simulink library "halin"  (R2021b)
settings: Solver=VariableStepAuto  StartTime=0.0  StopTime=10.0  RelTol=1e-3
undefined symbols (not defined in the file): KHAL_CAN1ABM1E2E_flg, KHAL_CAN1ESC1E2E_flg, KHAL_CAN1ESC5E2E_flg, KHAL_CAN1ESC7E2E_flg, KHAL_CAN1FCM2E2E_flg, KHAL_CAN1FCM3E2E_flg, KHAL_CAN1FCM4E2E_flg, KHAL_CAN3BMS1E2E_flg, KHAL_CAN3BMS6E2E_flg, KHAL_CAN3CCU1E2E_flg, KHAL_CAN3CCU2E2E_flg, KHAL_CAN3MCUF1E2E_flg, KHAL_CAN3MCUR1E2E_flg, KHAL_CAN3Shifter1E2E_flg, TRUE
libraries: simulink x420, FVT_lib x149, hcu_lib x49
(part 4 of 14)

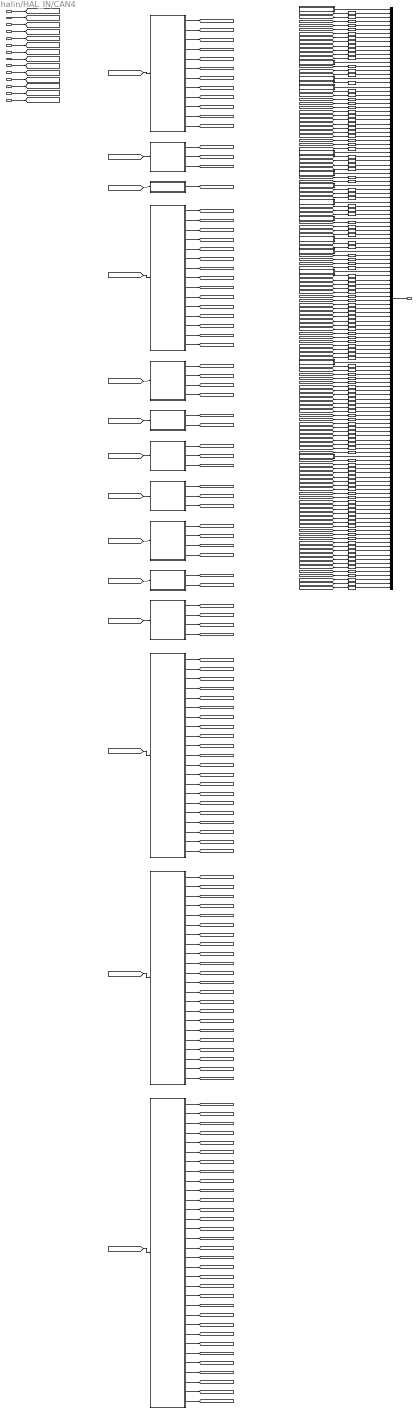
== system halin/HAL_IN/CAN4 ==
  DT_CAN4_SG_DKC1 : Inport
  DT_CAN4_SG_DKC2 : Inport  Port=2
  DT_CAN4_SG_GW_ZDR_PTG1 : Inport  Port=3
  DT_CAN4_SG_GW_ZoneDR1 : Inport  Port=4
  DT_CAN4_SG_GW_ZoneDR2 : Inport  Port=5
  DT_CAN4_SG_GW_ZoneDR3 : Inport  Port=6
  DT_CAN4_SG_GW_ZoneDR4 : Inport  Port=7
  DT_CAN4_SG_GW_ZoneDR6 : Inport  Port=8
  DT_CAN4_SG_GW_ZoneFR1 : Inport  Port=9
  DT_CAN4_SG_GW_ZoneFR2 : Inport  Port=10
  DT_CAN4_SG_Zone_Dr_SCP : Inport  Port=11
  DT_CAN4_SG_Zone_Dr_THCM : Inport  Port=12
  DT_CAN4_SG_Zone_Dr_VCU : Inport  Port=13
  DT_CAN4_SG_Zone_Fr_THCM : Inport  Port=14
  DKC1 : Subsystem
  DKC2 : Subsystem
  GW_ZDR_PTG1 : Subsystem
  GW_ZoneDR1 : Subsystem
  GW_ZoneDR2 : Subsystem
  GW_ZoneDR3 : Subsystem
  GW_ZoneDR4 : Subsystem
  GW_ZoneDR6 : Subsystem
  GW_ZoneFR1 : Subsystem
  GW_ZoneFR2 : Subsystem
  UnitConverter{,1..8,10,15,17..18,20..22,26,39,50,52..53,55,57,59,61,63,65,67,69,71,73,76,79..81,90,92,94..96,98,100..105,107,109,111,113,115,117,119,121..125,127} (60 alike) : DataTypeConversion  OutDataTypeStr=uint8
  UnitConverter{27..28,35..38,40..44,47,51,54,56,58,60,62,64,66,68,70,72,74..75,77..78,85..86,88..89,91,97,99,106,108,110,112,114,116,118,120,126} (43 alike) : DataTypeConversion  OutDataTypeStr=single
  UnitConverter{9,11,16,19,23..25,29..34,45..46,48..49,82..84,87,93} (22 alike) : DataTypeConversion  OutDataTypeStr=boolean
  UnitConverter12 : DataTypeConversion  OutDataTypeStr=uint64
  UnitConverter13 : DataTypeConversion  OutDataTypeStr=uint64
  UnitConverter14 : DataTypeConversion  OutDataTypeStr=uint64
  VHAL_CANMsgInvalidDKC1_flg : Subsystem  AncestorBlock=FVT_lib/hal/MsgTimeoutJudge_CAN_AUTOSAR
      mask help: MeasumentTrigerEvent
      mask Display: fprintf('MsgTimeoutJudge_CAN\nAUTOSAR');
  VHAL_CANMsgInvalidDKC2_flg : Subsystem  AncestorBlock=FVT_lib/hal/MsgTimeoutJudge_CAN_AUTOSAR
      mask help: MeasumentTrigerEvent
      mask Display: fprintf('MsgTimeoutJudge_CAN\nAUTOSAR');
  VHAL_CANMsgInvalidGWZDRPTG1_flg : Subsystem  AncestorBlock=FVT_lib/hal/MsgTimeoutJudge_CAN_AUTOSAR
      mask help: MeasumentTrigerEvent
      mask Display: fprintf('MsgTimeoutJudge_CAN\nAUTOSAR');
  VHAL_CANMsgInvalidGWZoneDR1_flg : Subsystem  AncestorBlock=FVT_lib/hal/MsgTimeoutJudge_CAN_AUTOSAR
      mask help: MeasumentTrigerEvent
      mask Display: fprintf('MsgTimeoutJudge_CAN\nAUTOSAR');
  VHAL_CANMsgInvalidGWZoneDR2_flg : Subsystem  AncestorBlock=FVT_lib/hal/MsgTimeoutJudge_CAN_AUTOSAR
      mask help: MeasumentTrigerEvent
      mask Display: fprintf('MsgTimeoutJudge_CAN\nAUTOSAR');
  VHAL_CANMsgInvalidGWZoneDR3_flg : Subsystem  AncestorBlock=FVT_lib/hal/MsgTimeoutJudge_CAN_AUTOSAR
      mask help: MeasumentTrigerEvent
      mask Display: fprintf('MsgTimeoutJudge_CAN\nAUTOSAR');
  VHAL_CANMsgInvalidGWZoneDR4_flg : Subsystem  AncestorBlock=FVT_lib/hal/MsgTimeoutJudge_CAN_AUTOSAR
      mask help: MeasumentTrigerEvent
      mask Display: fprintf('MsgTimeoutJudge_CAN\nAUTOSAR');
  VHAL_CANMsgInvalidGWZoneDR6_flg : Subsystem  AncestorBlock=FVT_lib/hal/MsgTimeoutJudge_CAN_AUTOSAR
      mask help: MeasumentTrigerEvent
      mask Display: fprintf('MsgTimeoutJudge_CAN\nAUTOSAR');
  VHAL_CANMsgInvalidGWZoneFR1_flg : Subsystem  AncestorBlock=FVT_lib/hal/MsgTimeoutJudge_CAN_AUTOSAR
      mask help: MeasumentTrigerEvent
      mask Display: fprintf('MsgTimeoutJudge_CAN\nAUTOSAR');
  VHAL_CANMsgInvalidGWZoneFR2_flg : Subsystem  AncestorBlock=FVT_lib/hal/MsgTimeoutJudge_CAN_AUTOSAR
      mask help: MeasumentTrigerEvent
      mask Display: fprintf('MsgTimeoutJudge_CAN\nAUTOSAR');
  VHAL_CANMsgInvalidZoneDrSCP_flg : Subsystem  AncestorBlock=FVT_lib/hal/MsgTimeoutJudge_CAN_AUTOSAR
      mask help: MeasumentTrigerEvent
      mask Display: fprintf('MsgTimeoutJudge_CAN\nAUTOSAR');
  VHAL_CANMsgInvalidZoneDrTHCM_flg : Subsystem  AncestorBlock=FVT_lib/hal/MsgTimeoutJudge_CAN_AUTOSAR
      mask help: MeasumentTrigerEvent
      mask Display: fprintf('MsgTimeoutJudge_CAN\nAUTOSAR');
  VHAL_CANMsgInvalidZoneDrVCU_flg : Subsystem  AncestorBlock=FVT_lib/hal/MsgTimeoutJudge_CAN_AUTOSAR
      mask help: MeasumentTrigerEvent
      mask Display: fprintf('MsgTimeoutJudge_CAN\nAUTOSAR');
  VHAL_CANMsgInvalidZoneFrTHCM_flg : Subsystem  AncestorBlock=FVT_lib/hal/MsgTimeoutJudge_CAN_AUTOSAR
      mask help: MeasumentTrigerEvent
      mask Display: fprintf('MsgTimeoutJudge_CAN\nAUTOSAR');
  Zone_Dr_SCP : Subsystem
  Zone_Dr_THCM : Subsystem
  Zone_Dr_VCU : Subsystem
  Zone_Fr_THCM : Subsystem
  bus_creator : BusCreator  Inputs=142
  HAL_CAN4_outputs : Outport
  wires:
  DT_CAN4_SG_DKC1/1 -> [DT_CAN4_SG_DKC1]
  DT_CAN4_SG_DKC2/1 -> [DT_CAN4_SG_DKC2]
  DT_CAN4_SG_GW_ZDR_PTG1/1 -> [DT_CAN4_SG_GW_ZDR_PTG1]
  DT_CAN4_SG_GW_ZoneDR1/1 -> [DT_CAN4_SG_GW_ZoneDR1]
  DT_CAN4_SG_GW_ZoneDR2/1 -> [DT_CAN4_SG_GW_ZoneDR2]
  DT_CAN4_SG_GW_ZoneDR3/1 -> [DT_CAN4_SG_GW_ZoneDR3]
  DT_CAN4_SG_GW_ZoneDR4/1 -> [DT_CAN4_SG_GW_ZoneDR4]
  DT_CAN4_SG_GW_ZoneDR6/1 -> [DT_CAN4_SG_GW_ZoneDR6]
  DT_CAN4_SG_GW_ZoneFR1/1 -> [DT_CAN4_SG_GW_ZoneFR1]
  DT_CAN4_SG_GW_ZoneFR2/1 -> [DT_CAN4_SG_GW_ZoneFR2]
  DT_CAN4_SG_Zone_Dr_SCP/1 -> [DT_CAN4_SG_Zone_Dr_SCP]
  DT_CAN4_SG_Zone_Dr_THCM/1 -> [DT_CAN4_SG_Zone_Dr_THCM]
  DT_CAN4_SG_Zone_Dr_VCU/1 -> [DT_CAN4_SG_Zone_Dr_VCU]
  DT_CAN4_SG_Zone_Fr_THCM/1 -> [DT_CAN4_SG_Zone_Fr_THCM]
  [DT_CAN4_SG_DKC1] -> DKC1/1(DT_CAN4_SG_DKC1)
  [DT_CAN4_SG_DKC2] -> DKC2/1(DT_CAN4_SG_DKC2)
  [DT_CAN4_SG_GW_ZDR_PTG1] -> GW_ZDR_PTG1/1(DT_CAN4_SG_GW_ZDR_PTG1)
  [DT_CAN4_SG_GW_ZoneDR1] -> GW_ZoneDR1/1(DT_CAN4_SG_GW_ZoneDR1)
  [DT_CAN4_SG_GW_ZoneDR2] -> GW_ZoneDR2/1(DT_CAN4_SG_GW_ZoneDR2)
  [DT_CAN4_SG_GW_ZoneDR3] -> GW_ZoneDR3/1(DT_CAN4_SG_GW_ZoneDR3)
  [DT_CAN4_SG_GW_ZoneDR4] -> GW_ZoneDR4/1(DT_CAN4_SG_GW_ZoneDR4)
  [DT_CAN4_SG_GW_ZoneDR6] -> GW_ZoneDR6/1(DT_CAN4_SG_GW_ZoneDR6)
  [DT_CAN4_SG_GW_ZoneFR1] -> GW_ZoneFR1/1(DT_CAN4_SG_GW_ZoneFR1)
  [DT_CAN4_SG_GW_ZoneFR2] -> GW_ZoneFR2/1(DT_CAN4_SG_GW_ZoneFR2)
  [DT_CAN4_SG_Zone_Dr_SCP] -> Zone_Dr_SCP/1(DT_CAN4_SG_Zone_Dr_SCP)
  [DT_CAN4_SG_Zone_Dr_THCM] -> Zone_Dr_THCM/1(DT_CAN4_SG_Zone_Dr_THCM)
  [DT_CAN4_SG_Zone_Dr_VCU] -> Zone_Dr_VCU/1(DT_CAN4_SG_Zone_Dr_VCU)
  [DT_CAN4_SG_Zone_Fr_THCM] -> Zone_Fr_THCM/1(DT_CAN4_SG_Zone_Fr_THCM)
  bus_creator/1 -> HAL_CAN4_outputs/1
  VHAL_CANMsgInvalidDKC1_flg/1(Out) -> bus_creator/1
  DKC1/1(VHAL_DKCReVehData_enum) -> [VHAL_DKCReVehData_enum]
  UnitConverter/1 -> bus_creator/2  "VHAL_DKCReVehData_enum"
  [VHAL_DKCReVehData_enum] -> UnitConverter/1
  DKC1/2(VHAL_DKCRemotePW_enum) -> [VHAL_DKCRemotePW_enum]
  UnitConverter1/1 -> bus_creator/3  "VHAL_DKCRemotePW_enum"
  [VHAL_DKCRemotePW_enum] -> UnitConverter1/1
  DKC1/3(VHAL_PCommandToBCM_enum) -> [VHAL_PCommandToBCM_enum]
  UnitConverter2/1 -> bus_creator/4  "VHAL_PCommandToBCM_enum"
  [VHAL_PCommandToBCM_enum] -> UnitConverter2/1
  DKC1/4(VHAL_PCommandToPTG_enum) -> [VHAL_PCommandToPTG_enum]
  UnitConverter3/1 -> bus_creator/5  "VHAL_PCommandToPTG_enum"
  [VHAL_PCommandToPTG_enum] -> UnitConverter3/1
  DKC1/5(VHAL_PDKeyAreaLockUnlock_enum) -> [VHAL_PDKeyAreaLockUnlock_enum]
  UnitConverter4/1 -> bus_creator/6  "VHAL_PDKeyAreaLockUnlock_enum"
  [VHAL_PDKeyAreaLockUnlock_enum] -> UnitConverter4/1
  DKC1/6(VHAL_PDKeyAreaPS_enum) -> [VHAL_PDKeyAreaPS_enum]
  UnitConverter5/1 -> bus_creator/7  "VHAL_PDKeyAreaPS_enum"
  [VHAL_PDKeyAreaPS_enum] -> UnitConverter5/1
  DKC1/7(VHAL_PDKeyAreaPTG_enum) -> [VHAL_PDKeyAreaPTG_enum]
  UnitConverter6/1 -> bus_creator/8  "VHAL_PDKeyAreaPTG_enum"
  [VHAL_PDKeyAreaPTG_enum] -> UnitConverter6/1
  DKC1/8(VHAL_PDKeyWelcome_enum) -> [VHAL_PDKeyWelcome_enum]
  UnitConverter7/1 -> bus_creator/9  "VHAL_PDKeyWelcome_enum"
  [VHAL_PDKeyWelcome_enum] -> UnitConverter7/1
  DKC1/9(VHAL_PDkeyShowIVI_enum) -> [VHAL_PDkeyShowIVI_enum]
  UnitConverter8/1 -> bus_creator/10  "VHAL_PDkeyShowIVI_enum"
  [VHAL_PDkeyShowIVI_enum] -> UnitConverter8/1
  DKC1/10(VHAL_PKeyMiss_flg) -> [VHAL_PKeyMiss_flg]
  UnitConverter9/1 -> bus_creator/11  "VHAL_PKeyMiss_flg"
  [VHAL_PKeyMiss_flg] -> UnitConverter9/1
  DKC1/11(VHAL_PKeyMode_enum) -> [VHAL_PKeyMode_enum]
  UnitConverter10/1 -> bus_creator/12  "VHAL_PKeyMode_enum"
  [VHAL_PKeyMode_enum] -> UnitConverter10/1
  DKC1/12(VHAL_PUIDLowPower_flg) -> [VHAL_PUIDLowPower_flg]
  UnitConverter11/1 -> bus_creator/13  "VHAL_PUIDLowPower_flg"
  [VHAL_PUIDLowPower_flg] -> UnitConverter11/1
  VHAL_CANMsgInvalidDKC2_flg/1(Out) -> bus_creator/14
  DKC2/1(VHAL_EncryptionDATA063_enum) -> [VHAL_EncryptionDATA063_enum]
  UnitConverter12/1 -> bus_creator/15  "VHAL_EncryptionDATA063_enum"
  [VHAL_EncryptionDATA063_enum] -> UnitConverter12/1
  DKC2/2(VHAL_EncryptionDATA64127_enum) -> [VHAL_EncryptionDATA64127_enum]
  UnitConverter13/1 -> bus_creator/16  "VHAL_EncryptionDATA64127_enum"
  [VHAL_EncryptionDATA64127_enum] -> UnitConverter13/1
  DKC2/3(VHAL_RandomNumberX_enum) -> [VHAL_RandomNumberX_enum]
  UnitConverter14/1 -> bus_creator/17  "VHAL_RandomNumberX_enum"
  [VHAL_RandomNumberX_enum] -> UnitConverter14/1
  VHAL_CANMsgInvalidGWZDRPTG1_flg/1(Out) -> bus_creator/18
  GW_ZDR_PTG1/1(VHAL_PTGRDILSta_enum) -> [VHAL_PTGRDILSta_enum]
  UnitConverter15/1 -> bus_creator/19  "VHAL_PTGRDILSta_enum"
  [VHAL_PTGRDILSta_enum] -> UnitConverter15/1
  VHAL_CANMsgInvalidGWZoneDR1_flg/1(Out) -> bus_creator/20
  GW_ZoneDR1/1(VHAL_CSWDimSw_flg) -> [VHAL_CSWDimSw_flg]
  UnitConverter16/1 -> bus_creator/21  "VHAL_CSWDimSw_flg"
  [VHAL_CSWDimSw_flg] -> UnitConverter16/1
  GW_ZoneDR1/2(VHAL_CSWFWasSwSta_enum) -> [VHAL_CSWFWasSwSta_enum]
  UnitConverter17/1 -> bus_creator/22  "VHAL_CSWFWasSwSta_enum"
  [VHAL_CSWFWasSwSta_enum] -> UnitConverter17/1
  GW_ZoneDR1/3(VHAL_CSWFWipSwSta_enum) -> [VHAL_CSWFWipSwSta_enum]
  UnitConverter18/1 -> bus_creator/23  "VHAL_CSWFWipSwSta_enum"
  [VHAL_CSWFWipSwSta_enum] -> UnitConverter18/1
  GW_ZoneDR1/4(VHAL_CSWPassSWSta_flg) -> [VHAL_CSWPassSWSta_flg]
  UnitConverter19/1 -> bus_creator/24  "VHAL_CSWPassSWSta_flg"
  [VHAL_CSWPassSWSta_flg] -> UnitConverter19/1
  GW_ZoneDR1/5(VHAL_CSWRWasSWSta_enum) -> [VHAL_CSWRWasSWSta_enum]
  UnitConverter20/1 -> bus_creator/25  "VHAL_CSWRWasSWSta_enum"
  [VHAL_CSWRWasSWSta_enum] -> UnitConverter20/1
  GW_ZoneDR1/6(VHAL_CSWRWipIntSwSta_enum) -> [VHAL_CSWRWipIntSwSta_enum]
  UnitConverter21/1 -> bus_creator/26  "VHAL_CSWRWipIntSwSta_enum"
  [VHAL_CSWRWipIntSwSta_enum] -> UnitConverter21/1
  GW_ZoneDR1/7(VHAL_CSWTurnSwSta_enum) -> [VHAL_CSWTurnSwSta_enum]
  UnitConverter22/1 -> bus_creator/27  "VHAL_CSWTurnSwSta_enum"
  [VHAL_CSWTurnSwSta_enum] -> UnitConverter22/1
  GW_ZoneDR1/8(VHAL_DrLockSta_flg) -> [VHAL_DrLockSta_flg]
  UnitConverter23/1 -> bus_creator/28  "VHAL_DrLockSta_flg"
  [VHAL_DrLockSta_flg] -> UnitConverter23/1
  GW_ZoneDR1/9(VHAL_MIRRORFOLDSW_flg) -> [VHAL_MIRRORFOLDSW_flg]
  UnitConverter24/1 -> bus_creator/29  "VHAL_MIRRORFOLDSW_flg"
  [VHAL_MIRRORFOLDSW_flg] -> UnitConverter24/1
  GW_ZoneDR1/10(VHAL_RLSLampSta_flg) -> [VHAL_RLSLampSta_flg]
  UnitConverter25/1 -> bus_creator/30  "VHAL_RLSLampSta_flg"
  [VHAL_RLSLampSta_flg] -> UnitConverter25/1
  GW_ZoneDR1/11(VHAL_RLSRainSnrWiperCmd_enum) -> [VHAL_RLSRainSnrWiperCmd_enum]
  UnitConverter26/1 -> bus_creator/31  "VHAL_RLSRainSnrWiperCmd_enum"
  [VHAL_RLSRainSnrWiperCmd_enum] -> UnitConverter26/1
  GW_ZoneDR1/12(VHAL_RLTurnLampC_mA) -> [VHAL_RLTurnLampC_mA]
  UnitConverter27/1 -> bus_creator/32  "VHAL_RLTurnLampC_mA"
  [VHAL_RLTurnLampC_mA] -> UnitConverter27/1
  GW_ZoneDR1/13(VHAL_RRTurnLampC_mA) -> [VHAL_RRTurnLampC_mA]
  UnitConverter28/1 -> bus_creator/33  "VHAL_RRTurnLampC_mA"
  [VHAL_RRTurnLampC_mA] -> UnitConverter28/1
  GW_ZoneDR1/14(VHAL_RWiperAS_flg) -> [VHAL_RWiperAS_flg]
  UnitConverter29/1 -> bus_creator/34  "VHAL_RWiperAS_flg"
  [VHAL_RWiperAS_flg] -> UnitConverter29/1
  GW_ZoneDR1/15(VHAL_RWiperProtection_flg) -> [VHAL_RWiperProtection_flg]
  UnitConverter30/1 -> bus_creator/35  "VHAL_RWiperProtection_flg"
  [VHAL_RWiperProtection_flg] -> UnitConverter30/1
  VHAL_CANMsgInvalidGWZoneDR2_flg/1(Out) -> bus_creator/36
  GW_ZoneDR2/1(VHAL_SWCCANCELSta_flg) -> [VHAL_SWCCANCELSta_flg]
  UnitConverter31/1 -> bus_creator/37  "VHAL_SWCCANCELSta_flg"
  [VHAL_SWCCANCELSta_flg] -> UnitConverter31/1
  GW_ZoneDR2/2(VHAL_SWCResUpSta_flg) -> [VHAL_SWCResUpSta_flg]
  UnitConverter32/1 -> bus_creator/38  "VHAL_SWCResUpSta_flg"
  [VHAL_SWCResUpSta_flg] -> UnitConverter32/1
  GW_ZoneDR2/3(VHAL_SWCSetdownSta_flg) -> [VHAL_SWCSetdownSta_flg]
  UnitConverter33/1 -> bus_creator/39  "VHAL_SWCSetdownSta_flg"
  [VHAL_SWCSetdownSta_flg] -> UnitConverter33/1
  GW_ZoneDR2/4(VHAL_SWCmodeSta_flg) -> [VHAL_SWCmodeSta_flg]
  UnitConverter34/1 -> bus_creator/40  "VHAL_SWCmodeSta_flg"
  [VHAL_SWCmodeSta_flg] -> UnitConverter34/1
  VHAL_CANMsgInvalidGWZoneDR3_flg/1(Out) -> bus_creator/41
  GW_ZoneDR3/1(VHAL_LDrvValWdwOpened_pct) -> [VHAL_LDrvValWdwOpened_pct]
  UnitConverter35/1 -> bus_creator/42  "VHAL_LDrvValWdwOpened_pct"
  [VHAL_LDrvValWdwOpened_pct] -> UnitConverter35/1
  GW_ZoneDR3/2(VHAL_LPasValWdwOpened_pct) -> [VHAL_LPasValWdwOpened_pct]
  UnitConverter36/1 -> bus_creator/43  "VHAL_LPasValWdwOpened_pct"
  [VHAL_LPasValWdwOpened_pct] -> UnitConverter36/1
  VHAL_CANMsgInvalidGWZoneDR4_flg/1(Out) -> bus_creator/44
  GW_ZoneDR4/1(VHAL_LRLDValWdwOpened_pct) -> [VHAL_LRLDValWdwOpened_pct]
  UnitConverter37/1 -> bus_creator/45  "VHAL_LRLDValWdwOpened_pct"
  [VHAL_LRLDValWdwOpened_pct] -> UnitConverter37/1
  GW_ZoneDR4/2(VHAL_LRRDValWdwOpened_pct) -> [VHAL_LRRDValWdwOpened_pct]
  UnitConverter38/1 -> bus_creator/46  "VHAL_LRRDValWdwOpened_pct"
  [VHAL_LRRDValWdwOpened_pct] -> UnitConverter38/1
  GW_ZoneDR4/3(VHAL_PTGInnerSW2_enum) -> [VHAL_PTGInnerSW2_enum]
  UnitConverter39/1 -> bus_creator/47  "VHAL_PTGInnerSW2_enum"
  [VHAL_PTGInnerSW2_enum] -> UnitConverter39/1
  VHAL_CANMsgInvalidGWZoneDR6_flg/1(Out) -> bus_creator/48
  GW_ZoneDR6/1(VHAL_FrntPTCRearLeActHeatPwr_W) -> [VHAL_FrntPTCRearLeActHeatPwr_W]
  UnitConverter40/1 -> bus_creator/49  "VHAL_FrntPTCRearLeActHeatPwr_W"
  [VHAL_FrntPTCRearLeActHeatPwr_W] -> UnitConverter40/1
  GW_ZoneDR6/2(VHAL_FrntPTCRearRiActHeatPwr_W) -> [VHAL_FrntPTCRearRiActHeatPwr_W]
  UnitConverter41/1 -> bus_creator/50  "VHAL_FrntPTCRearRiActHeatPwr_W"
  [VHAL_FrntPTCRearRiActHeatPwr_W] -> UnitConverter41/1
  GW_ZoneDR6/3(VHAL_FrntPTCRiActHeatPwr_W) -> [VHAL_FrntPTCRiActHeatPwr_W]
  UnitConverter42/1 -> bus_creator/51  "VHAL_FrntPTCRiActHeatPwr_W"
  [VHAL_FrntPTCRiActHeatPwr_W] -> UnitConverter42/1
  VHAL_CANMsgInvalidGWZoneFR1_flg/1(Out) -> bus_creator/52
  GW_ZoneFR1/1(VHAL_FLTurnLampC_mA) -> [VHAL_FLTurnLampC_mA]
  UnitConverter43/1 -> bus_creator/53  "VHAL_FLTurnLampC_mA"
  [VHAL_FLTurnLampC_mA] -> UnitConverter43/1
  GW_ZoneFR1/2(VHAL_FRTurnLampC_mA) -> [VHAL_FRTurnLampC_mA]
  UnitConverter44/1 -> bus_creator/54  "VHAL_FRTurnLampC_mA"
  [VHAL_FRTurnLampC_mA] -> UnitConverter44/1
  GW_ZoneFR1/3(VHAL_FWiperAS_flg) -> [VHAL_FWiperAS_flg]
  UnitConverter45/1 -> bus_creator/55  "VHAL_FWiperAS_flg"
  [VHAL_FWiperAS_flg] -> UnitConverter45/1
  GW_ZoneFR1/4(VHAL_FWiperProtection_flg) -> [VHAL_FWiperProtection_flg]
  UnitConverter46/1 -> bus_creator/56  "VHAL_FWiperProtection_flg"
  [VHAL_FWiperProtection_flg] -> UnitConverter46/1
  VHAL_CANMsgInvalidGWZoneFR2_flg/1(Out) -> bus_creator/57
  GW_ZoneFR2/1(VHAL_COMPStatorSpd_rpm) -> [VHAL_COMPStatorSpd_rpm]
  UnitConverter47/1 -> bus_creator/58  "VHAL_COMPStatorSpd_rpm"
  [VHAL_COMPStatorSpd_rpm] -> UnitConverter47/1
  GW_ZoneFR2/2(VHAL_CompProEN_flg) -> [VHAL_CompProEN_flg]
  UnitConverter48/1 -> bus_creator/59  "VHAL_CompProEN_flg"
  [VHAL_CompProEN_flg] -> UnitConverter48/1
  VHAL_CANMsgInvalidZoneDrSCP_flg/1(Out) -> bus_creator/60
  Zone_Dr_SCP/1(VHAL_DrSCPSysErrLmp_flg) -> [VHAL_DrSCPSysErrLmp_flg]
  UnitConverter49/1 -> bus_creator/61  "VHAL_DrSCPSysErrLmp_flg"
  [VHAL_DrSCPSysErrLmp_flg] -> UnitConverter49/1
  Zone_Dr_SCP/2(VHAL_RegenMode_enum) -> [VHAL_RegenMode_enum]
  UnitConverter50/1 -> bus_creator/62  "VHAL_RegenMode_enum"
  [VHAL_RegenMode_enum] -> UnitConverter50/1
  Zone_Dr_SCP/3(VHAL_SetSpd_kph) -> [VHAL_SetSpd_kph]
  UnitConverter51/1 -> bus_creator/63  "VHAL_SetSpd_kph"
  [VHAL_SetSpd_kph] -> UnitConverter51/1
  Zone_Dr_SCP/4(VHAL_ZoneSpdCtrlMode_enum) -> [VHAL_ZoneSpdCtrlMode_enum]
  UnitConverter52/1 -> bus_creator/64  "VHAL_ZoneSpdCtrlMode_enum"
  [VHAL_ZoneSpdCtrlMode_enum] -> UnitConverter52/1
  VHAL_CANMsgInvalidZoneDrTHCM_flg/1(Out) -> bus_creator/65
  Zone_Dr_THCM/1(VHAL_BlowerErr_enum) -> [VHAL_BlowerErr_enum]
  UnitConverter53/1 -> bus_creator/66  "VHAL_BlowerErr_enum"
  [VHAL_BlowerErr_enum] -> UnitConverter53/1
  Zone_Dr_THCM/2(VHAL_SolarL_W) -> [VHAL_SolarL_W]
  UnitConverter54/1 -> bus_creator/67  "VHAL_SolarL_W"
  [VHAL_SolarL_W] -> UnitConverter54/1
  Zone_Dr_THCM/3(VHAL_SolarLErr_enum) -> [VHAL_SolarLErr_enum]
  UnitConverter55/1 -> bus_creator/68  "VHAL_SolarLErr_enum"
  [VHAL_SolarLErr_enum] -> UnitConverter55/1
  Zone_Dr_THCM/4(VHAL_SolarR_W) -> [VHAL_SolarR_W]
  UnitConverter56/1 -> bus_creator/69  "VHAL_SolarR_W"
  [VHAL_SolarR_W] -> UnitConverter56/1
  Zone_Dr_THCM/5(VHAL_SolarRErr_enum) -> [VHAL_SolarRErr_enum]
  UnitConverter57/1 -> bus_creator/70  "VHAL_SolarRErr_enum"
  [VHAL_SolarRErr_enum] -> UnitConverter57/1
  Zone_Dr_THCM/6(VHAL_TFaceL_C) -> [VHAL_TFaceL_C]
  UnitConverter58/1 -> bus_creator/71  "VHAL_TFaceL_C"
  [VHAL_TFaceL_C] -> UnitConverter58/1
  Zone_Dr_THCM/7(VHAL_TFaceLErr_enum) -> [VHAL_TFaceLErr_enum]
  UnitConverter59/1 -> bus_creator/72  "VHAL_TFaceLErr_enum"
  [VHAL_TFaceLErr_enum] -> UnitConverter59/1
  Zone_Dr_THCM/8(VHAL_TFaceR_C) -> [VHAL_TFaceR_C]
  UnitConverter60/1 -> bus_creator/73  "VHAL_TFaceR_C"
  [VHAL_TFaceR_C] -> UnitConverter60/1
  Zone_Dr_THCM/9(VHAL_TFaceRErr_enum) -> [VHAL_TFaceRErr_enum]
  UnitConverter61/1 -> bus_creator/74  "VHAL_TFaceRErr_enum"
  [VHAL_TFaceRErr_enum] -> UnitConverter61/1
  Zone_Dr_THCM/10(VHAL_TFaceRr_C) -> [VHAL_TFaceRr_C]
  UnitConverter62/1 -> bus_creator/75  "VHAL_TFaceRr_C"
  [VHAL_TFaceRr_C] -> UnitConverter62/1
  Zone_Dr_THCM/11(VHAL_TFaceRrErr_enum) -> [VHAL_TFaceRrErr_enum]
  UnitConverter63/1 -> bus_creator/76  "VHAL_TFaceRrErr_enum"
  [VHAL_TFaceRrErr_enum] -> UnitConverter63/1
  Zone_Dr_THCM/12(VHAL_TFootL_C) -> [VHAL_TFootL_C]
  UnitConverter64/1 -> bus_creator/77  "VHAL_TFootL_C"
  [VHAL_TFootL_C] -> UnitConverter64/1
  Zone_Dr_THCM/13(VHAL_TFootLErr_enum) -> [VHAL_TFootLErr_enum]
  UnitConverter65/1 -> bus_creator/78  "VHAL_TFootLErr_enum"
  [VHAL_TFootLErr_enum] -> UnitConverter65/1
  Zone_Dr_THCM/14(VHAL_TFootR_C) -> [VHAL_TFootR_C]
  UnitConverter66/1 -> bus_creator/79  "VHAL_TFootR_C"
  [VHAL_TFootR_C] -> UnitConverter66/1
  Zone_Dr_THCM/15(VHAL_TFootRErr_enum) -> [VHAL_TFootRErr_enum]
  UnitConverter67/1 -> bus_creator/80  "VHAL_TFootRErr_enum"
  [VHAL_TFootRErr_enum] -> UnitConverter67/1
  Zone_Dr_THCM/16(VHAL_TFootRr_C) -> [VHAL_TFootRr_C]
  UnitConverter68/1 -> bus_creator/81  "VHAL_TFootRr_C"
  [VHAL_TFootRr_C] -> UnitConverter68/1
  Zone_Dr_THCM/17(VHAL_TFootRrErr_enum) -> [VHAL_TFootRrErr_enum]
  UnitConverter69/1 -> bus_creator/82  "VHAL_TFootRrErr_enum"
  [VHAL_TFootRrErr_enum] -> UnitConverter69/1
  Zone_Dr_THCM/18(VHAL_Tevap_C) -> [VHAL_Tevap_C]
  UnitConverter70/1 -> bus_creator/83  "VHAL_Tevap_C"
  [VHAL_Tevap_C] -> UnitConverter70/1
  Zone_Dr_THCM/19(VHAL_TevapErr_enum) -> [VHAL_TevapErr_enum]
  UnitConverter71/1 -> bus_creator/84  "VHAL_TevapErr_enum"
  [VHAL_TevapErr_enum] -> UnitConverter71/1
  Zone_Dr_THCM/20(VHAL_Tincar_C) -> [VHAL_Tincar_C]
  UnitConverter72/1 -> bus_creator/85  "VHAL_Tincar_C"
  [VHAL_Tincar_C] -> UnitConverter72/1
  Zone_Dr_THCM/21(VHAL_TincarErr_enum) -> [VHAL_TincarErr_enum]
  UnitConverter73/1 -> bus_creator/86  "VHAL_TincarErr_enum"
  [VHAL_TincarErr_enum] -> UnitConverter73/1
  VHAL_CANMsgInvalidZoneDrVCU_flg/1(Out) -> bus_creator/87
  Zone_Dr_VCU/1(VHAL_DrAuBoxPwrN1Curr_A) -> [VHAL_DrAuBoxPwrN1Curr_A]
  UnitConverter74/1 -> bus_creator/88  "VHAL_DrAuBoxPwrN1Curr_A"
  [VHAL_DrAuBoxPwrN1Curr_A] -> UnitConverter74/1
  Zone_Dr_VCU/2(VHAL_DrAuBoxPwrN2Curr_A) -> [VHAL_DrAuBoxPwrN2Curr_A]
  UnitConverter75/1 -> bus_creator/89  "VHAL_DrAuBoxPwrN2Curr_A"
  [VHAL_DrAuBoxPwrN2Curr_A] -> UnitConverter75/1
  Zone_Dr_VCU/3(VHAL_DrColumnSWFault_enum) -> [VHAL_DrColumnSWFault_enum]
  UnitConverter76/1 -> bus_creator/90  "VHAL_DrColumnSWFault_enum"
  [VHAL_DrColumnSWFault_enum] -> UnitConverter76/1
  Zone_Dr_VCU/4(VHAL_DrCtrlBDVolt_V) -> [VHAL_DrCtrlBDVolt_V]
  UnitConverter77/1 -> bus_creator/91  "VHAL_DrCtrlBDVolt_V"
  [VHAL_DrCtrlBDVolt_V] -> UnitConverter77/1
  Zone_Dr_VCU/5(VHAL_DrCtrlTemp_C) -> [VHAL_DrCtrlTemp_C]
  UnitConverter78/1 -> bus_creator/92  "VHAL_DrCtrlTemp_C"
  [VHAL_DrCtrlTemp_C] -> UnitConverter78/1
  Zone_Dr_VCU/6(VHAL_DrEOBDFault_enum) -> [VHAL_DrEOBDFault_enum]
  UnitConverter79/1 -> bus_creator/93  "VHAL_DrEOBDFault_enum"
  [VHAL_DrEOBDFault_enum] -> UnitConverter79/1
  Zone_Dr_VCU/7(VHAL_DrIVIFault_enum) -> [VHAL_DrIVIFault_enum]
  UnitConverter80/1 -> bus_creator/94  "VHAL_DrIVIFault_enum"
  [VHAL_DrIVIFault_enum] -> UnitConverter80/1
  Zone_Dr_VCU/8(VHAL_DrInfoFault_enum) -> [VHAL_DrInfoFault_enum]
  UnitConverter81/1 -> bus_creator/95  "VHAL_DrInfoFault_enum"
  [VHAL_DrInfoFault_enum] -> UnitConverter81/1
  Zone_Dr_VCU/9(VHAL_DrPMMLVOutPErrLmp_flg) -> [VHAL_DrPMMLVOutPErrLmp_flg]
  UnitConverter82/1 -> bus_creator/96  "VHAL_DrPMMLVOutPErrLmp_flg"
  [VHAL_DrPMMLVOutPErrLmp_flg] -> UnitConverter82/1
  Zone_Dr_VCU/10(VHAL_DrPMMLimpHomeActReq_flg) -> [VHAL_DrPMMLimpHomeActReq_flg]
  UnitConverter83/1 -> bus_creator/97  "VHAL_DrPMMLimpHomeActReq_flg"
  [VHAL_DrPMMLimpHomeActReq_flg] -> UnitConverter83/1
  Zone_Dr_VCU/11(VHAL_DrPMMSysErrLmp_flg) -> [VHAL_DrPMMSysErrLmp_flg]
  UnitConverter84/1 -> bus_creator/98  "VHAL_DrPMMSysErrLmp_flg"
  [VHAL_DrPMMSysErrLmp_flg] -> UnitConverter84/1
  Zone_Dr_VCU/12(VHAL_DrPowerTemp1_C) -> [VHAL_DrPowerTemp1_C]
  UnitConverter85/1 -> bus_creator/99  "VHAL_DrPowerTemp1_C"
  [VHAL_DrPowerTemp1_C] -> UnitConverter85/1
  Zone_Dr_VCU/13(VHAL_DrPowerTemp2_C) -> [VHAL_DrPowerTemp2_C]
  UnitConverter86/1 -> bus_creator/100  "VHAL_DrPowerTemp2_C"
  [VHAL_DrPowerTemp2_C] -> UnitConverter86/1
  Zone_Dr_VCU/14(VHAL_DrPwrInformationSta_flg) -> [VHAL_DrPwrInformationSta_flg]
  UnitConverter87/1 -> bus_creator/101  "VHAL_DrPwrInformationSta_flg"
  [VHAL_DrPwrInformationSta_flg] -> UnitConverter87/1
  Zone_Dr_VCU/15(VHAL_DrPwrONA1Curr_A) -> [VHAL_DrPwrONA1Curr_A]
  UnitConverter88/1 -> bus_creator/102  "VHAL_DrPwrONA1Curr_A"
  [VHAL_DrPwrONA1Curr_A] -> UnitConverter88/1
  Zone_Dr_VCU/16(VHAL_DrPwrONA2Curr_A) -> [VHAL_DrPwrONA2Curr_A]
  UnitConverter89/1 -> bus_creator/103  "VHAL_DrPwrONA2Curr_A"
  [VHAL_DrPwrONA2Curr_A] -> UnitConverter89/1
  Zone_Dr_VCU/17(VHAL_DrPwrSta_enum) -> [VHAL_DrPwrSta_enum]
  UnitConverter90/1 -> bus_creator/104  "VHAL_DrPwrSta_enum"
  [VHAL_DrPwrSta_enum] -> UnitConverter90/1
  Zone_Dr_VCU/18(VHAL_DrPwrStdbyACurr_A) -> [VHAL_DrPwrStdbyACurr_A]
  UnitConverter91/1 -> bus_creator/105  "VHAL_DrPwrStdbyACurr_A"
  [VHAL_DrPwrStdbyACurr_A] -> UnitConverter91/1
  Zone_Dr_VCU/19(VHAL_DrPwrWindowECUFault_enum) -> [VHAL_DrPwrWindowECUFault_enum]
  UnitConverter92/1 -> bus_creator/106  "VHAL_DrPwrWindowECUFault_enum"
  [VHAL_DrPwrWindowECUFault_enum] -> UnitConverter92/1
  Zone_Dr_VCU/20(VHAL_DrStdAErrSta_flg) -> [VHAL_DrStdAErrSta_flg]
  UnitConverter93/1 -> bus_creator/107  "VHAL_DrStdAErrSta_flg"
  [VHAL_DrStdAErrSta_flg] -> UnitConverter93/1
  Zone_Dr_VCU/21(VHAL_DrTHCMFault_enum) -> [VHAL_DrTHCMFault_enum]
  UnitConverter94/1 -> bus_creator/108  "VHAL_DrTHCMFault_enum"
  [VHAL_DrTHCMFault_enum] -> UnitConverter94/1
  Zone_Dr_VCU/22(VHAL_ZoneDrMalfunLevel_enum) -> [VHAL_ZoneDrMalfunLevel_enum]
  UnitConverter95/1 -> bus_creator/109  "VHAL_ZoneDrMalfunLevel_enum"
  [VHAL_ZoneDrMalfunLevel_enum] -> UnitConverter95/1
  VHAL_CANMsgInvalidZoneFrTHCM_flg/1(Out) -> bus_creator/110
  Zone_Fr_THCM/1(VHAL_AGSErr_enum) -> [VHAL_AGSErr_enum]
  UnitConverter96/1 -> bus_creator/111  "VHAL_AGSErr_enum"
  [VHAL_AGSErr_enum] -> UnitConverter96/1
  Zone_Fr_THCM/2(VHAL_BatInTemp_C) -> [VHAL_BatInTemp_C]
  UnitConverter97/1 -> bus_creator/112  "VHAL_BatInTemp_C"
  [VHAL_BatInTemp_C] -> UnitConverter97/1
  Zone_Fr_THCM/3(VHAL_BatInTempErr_enum) -> [VHAL_BatInTempErr_enum]
  UnitConverter98/1 -> bus_creator/113  "VHAL_BatInTempErr_enum"
  [VHAL_BatInTempErr_enum] -> UnitConverter98/1
  Zone_Fr_THCM/4(VHAL_BatOutTemp_C) -> [VHAL_BatOutTemp_C]
  UnitConverter99/1 -> bus_creator/114  "VHAL_BatOutTemp_C"
  [VHAL_BatOutTemp_C] -> UnitConverter99/1
  Zone_Fr_THCM/5(VHAL_COMPErr_enum) -> [VHAL_COMPErr_enum]
  UnitConverter100/1 -> bus_creator/115  "VHAL_COMPErr_enum"
  [VHAL_COMPErr_enum] -> UnitConverter100/1
  Zone_Fr_THCM/6(VHAL_EACProtectEnable_enum) -> [VHAL_EACProtectEnable_enum]
  UnitConverter101/1 -> bus_creator/116  "VHAL_EACProtectEnable_enum"
  [VHAL_EACProtectEnable_enum] -> UnitConverter101/1
  Zone_Fr_THCM/7(VHAL_EWP3Err_enum) -> [VHAL_EWP3Err_enum]
  UnitConverter102/1 -> bus_creator/117  "VHAL_EWP3Err_enum"
  [VHAL_EWP3Err_enum] -> UnitConverter102/1
  Zone_Fr_THCM/8(VHAL_EXV1Err_enum) -> [VHAL_EXV1Err_enum]
  UnitConverter103/1 -> bus_creator/118  "VHAL_EXV1Err_enum"
  [VHAL_EXV1Err_enum] -> UnitConverter103/1
  Zone_Fr_THCM/9(VHAL_EXV2Err_enum) -> [VHAL_EXV2Err_enum]
  UnitConverter104/1 -> bus_creator/119  "VHAL_EXV2Err_enum"
  [VHAL_EXV2Err_enum] -> UnitConverter104/1
  Zone_Fr_THCM/10(VHAL_FanErr_enum) -> [VHAL_FanErr_enum]
  UnitConverter105/1 -> bus_creator/120  "VHAL_FanErr_enum"
  [VHAL_FanErr_enum] -> UnitConverter105/1
  Zone_Fr_THCM/11(VHAL_MotorInTemp_C) -> [VHAL_MotorInTemp_C]
  UnitConverter106/1 -> bus_creator/121  "VHAL_MotorInTemp_C"
  [VHAL_MotorInTemp_C] -> UnitConverter106/1
  Zone_Fr_THCM/12(VHAL_MotorInTempErr_enum) -> [VHAL_MotorInTempErr_enum]
  UnitConverter107/1 -> bus_creator/122  "VHAL_MotorInTempErr_enum"
  [VHAL_MotorInTempErr_enum] -> UnitConverter107/1
  Zone_Fr_THCM/13(VHAL_MotorOutTemp_C) -> [VHAL_MotorOutTemp_C]
  UnitConverter108/1 -> bus_creator/123  "VHAL_MotorOutTemp_C"
  [VHAL_MotorOutTemp_C] -> UnitConverter108/1
  Zone_Fr_THCM/14(VHAL_MotorOutTempErr_enum) -> [VHAL_MotorOutTempErr_enum]
  UnitConverter109/1 -> bus_creator/124  "VHAL_MotorOutTempErr_enum"
  [VHAL_MotorOutTempErr_enum] -> UnitConverter109/1
  Zone_Fr_THCM/15(VHAL_PTHighP_KPa) -> [VHAL_PTHighP_KPa]
  UnitConverter110/1 -> bus_creator/125  "VHAL_PTHighP_KPa"
  [VHAL_PTHighP_KPa] -> UnitConverter110/1
  Zone_Fr_THCM/16(VHAL_PTHighPErr_enum) -> [VHAL_PTHighPErr_enum]
  UnitConverter111/1 -> bus_creator/126  "VHAL_PTHighPErr_enum"
  [VHAL_PTHighPErr_enum] -> UnitConverter111/1
  Zone_Fr_THCM/17(VHAL_PTHighTact_C) -> [VHAL_PTHighTact_C]
  UnitConverter112/1 -> bus_creator/127  "VHAL_PTHighTact_C"
  [VHAL_PTHighTact_C] -> UnitConverter112/1
  Zone_Fr_THCM/18(VHAL_PTHighTactErr_enum) -> [VHAL_PTHighTactErr_enum]
  UnitConverter113/1 -> bus_creator/128  "VHAL_PTHighTactErr_enum"
  [VHAL_PTHighTactErr_enum] -> UnitConverter113/1
  Zone_Fr_THCM/19(VHAL_PTLowP1_KPa) -> [VHAL_PTLowP1_KPa]
  UnitConverter114/1 -> bus_creator/129  "VHAL_PTLowP1_KPa"
  [VHAL_PTLowP1_KPa] -> UnitConverter114/1
  Zone_Fr_THCM/20(VHAL_PTLowP1Err_enum) -> [VHAL_PTLowP1Err_enum]
  UnitConverter115/1 -> bus_creator/130  "VHAL_PTLowP1Err_enum"
  [VHAL_PTLowP1Err_enum] -> UnitConverter115/1
  Zone_Fr_THCM/21(VHAL_PTLowP2_KPa) -> [VHAL_PTLowP2_KPa]
  UnitConverter116/1 -> bus_creator/131  "VHAL_PTLowP2_KPa"
  [VHAL_PTLowP2_KPa] -> UnitConverter116/1
  Zone_Fr_THCM/22(VHAL_PTLowP2Err_enum) -> [VHAL_PTLowP2Err_enum]
  UnitConverter117/1 -> bus_creator/132  "VHAL_PTLowP2Err_enum"
  [VHAL_PTLowP2Err_enum] -> UnitConverter117/1
  Zone_Fr_THCM/23(VHAL_PTLowT1_C) -> [VHAL_PTLowT1_C]
  UnitConverter118/1 -> bus_creator/133  "VHAL_PTLowT1_C"
  [VHAL_PTLowT1_C] -> UnitConverter118/1
  Zone_Fr_THCM/24(VHAL_PTLowT1Err_enum) -> [VHAL_PTLowT1Err_enum]
  UnitConverter119/1 -> bus_creator/134  "VHAL_PTLowT1Err_enum"
  [VHAL_PTLowT1Err_enum] -> UnitConverter119/1
  Zone_Fr_THCM/25(VHAL_PTLowT2_C) -> [VHAL_PTLowT2_C]
  UnitConverter120/1 -> bus_creator/135  "VHAL_PTLowT2_C"
  [VHAL_PTLowT2_C] -> UnitConverter120/1
  Zone_Fr_THCM/26(VHAL_PTLowT2Err_enum) -> [VHAL_PTLowT2Err_enum]
  UnitConverter121/1 -> bus_creator/136  "VHAL_PTLowT2Err_enum"
  [VHAL_PTLowT2Err_enum] -> UnitConverter121/1
  Zone_Fr_THCM/27(VHAL_SOTXVErr_enum) -> [VHAL_SOTXVErr_enum]
  UnitConverter122/1 -> bus_creator/137  "VHAL_SOTXVErr_enum"
  [VHAL_SOTXVErr_enum] -> UnitConverter122/1
  Zone_Fr_THCM/28(VHAL_SOV1Err_enum) -> [VHAL_SOV1Err_enum]
  UnitConverter123/1 -> bus_creator/138  "VHAL_SOV1Err_enum"
  [VHAL_SOV1Err_enum] -> UnitConverter123/1
  Zone_Fr_THCM/29(VHAL_SOV2Err_enum) -> [VHAL_SOV2Err_enum]
  UnitConverter124/1 -> bus_creator/139  "VHAL_SOV2Err_enum"
  [VHAL_SOV2Err_enum] -> UnitConverter124/1
  Zone_Fr_THCM/30(VHAL_SOV3Err_enum) -> [VHAL_SOV3Err_enum]
  UnitConverter125/1 -> bus_creator/140  "VHAL_SOV3Err_enum"
  [VHAL_SOV3Err_enum] -> UnitConverter125/1
  Zone_Fr_THCM/31(VHAL_Tamb_C) -> [VHAL_Tamb_C]
  UnitConverter126/1 -> bus_creator/141  "VHAL_Tamb_C"
  [VHAL_Tamb_C] -> UnitConverter126/1
  Zone_Fr_THCM/32(VHAL_TambErr_enum) -> [VHAL_TambErr_enum]
  UnitConverter127/1 -> bus_creator/142  "VHAL_TambErr_enum"
  [VHAL_TambErr_enum] -> UnitConverter127/1

== system halin/HAL_IN/CAN5 ==
  DT_CAN5_SG_TBOX1 : Inport
  TBOX1 : Subsystem
  UnitConverter : DataTypeConversion  OutDataTypeStr=single
  UnitConverter1 : DataTypeConversion  OutDataTypeStr=uint8
  UnitConverter2 : DataTypeConversion  OutDataTypeStr=uint16
  UnitConverter3 : DataTypeConversion  OutDataTypeStr=uint8
  UnitConverter4 : DataTypeConversion  OutDataTypeStr=single
  UnitConverter5 : DataTypeConversion  OutDataTypeStr=boolean
  VHAL_CANMsgInvalidTBOX1_flg : Subsystem  AncestorBlock=FVT_lib/hal/MsgTimeoutJudge_CAN_AUTOSAR
      mask help: MeasumentTrigerEvent
      mask Display: fprintf('MsgTimeoutJudge_CAN\nAUTOSAR');
  bus_creator : BusCreator  Inputs=7
  HAL_CAN5_outputs : Outport
  wires:
  DT_CAN5_SG_TBOX1/1 -> [DT_CAN5_SG_TBOX1]
  [DT_CAN5_SG_TBOX1] -> TBOX1/1(DT_CAN5_SG_TBOX1)
  bus_creator/1 -> HAL_CAN5_outputs/1
  VHAL_CANMsgInvalidTBOX1_flg/1(Out) -> bus_creator/1
  TBOX1/1(VHAL_PowerOffTSet_cnt) -> [VHAL_PowerOffTSet_cnt]
  UnitConverter/1 -> bus_creator/2  "VHAL_PowerOffTSet_cnt"
  [VHAL_PowerOffTSet_cnt] -> UnitConverter/1
  TBOX1/2(VHAL_ReOutsideMirror_enum) -> [VHAL_ReOutsideMirror_enum]
  UnitConverter1/1 -> bus_creator/3  "VHAL_ReOutsideMirror_enum"
  [VHAL_ReOutsideMirror_enum] -> UnitConverter1/1
  TBOX1/3(VHAL_ReDoorLock_enum) -> [VHAL_ReDoorLock_enum]
  UnitConverter2/1 -> bus_creator/4  "VHAL_ReDoorLock_enum"
  [VHAL_ReDoorLock_enum] -> UnitConverter2/1
  TBOX1/4(VHAL_RePwrReqTbox_enum) -> [VHAL_RePwrReqTbox_enum]
  UnitConverter3/1 -> bus_creator/5  "VHAL_RePwrReqTbox_enum"
  [VHAL_RePwrReqTbox_enum] -> UnitConverter3/1
  TBOX1/5(VHAL_RemoteACTemp_C) -> [VHAL_RemoteACTemp_C]
  UnitConverter4/1 -> bus_creator/6  "VHAL_RemoteACTemp_C"
  [VHAL_RemoteACTemp_C] -> UnitConverter4/1
  TBOX1/6(VHAL_RemoteAutoReq_flg) -> [VHAL_RemoteAutoReq_flg]
  UnitConverter5/1 -> bus_creator/7  "VHAL_RemoteAutoReq_flg"
  [VHAL_RemoteAutoReq_flg] -> UnitConverter5/1

== system halin/HAL_IN/CAN1/ABM1 ==
  DT_CAN1_SG_ABM1 : Inport
  0xe4 : Constant  Value=0xe4
  0xf2 : Constant  Value=0xf2
  AirBagFailCmd : Subsystem
  BitwiseAND{,1..11} (12 alike) : simulink/Logic and Bit Operations/Bitwise Operator  logicop=AND  UseBitMask=on  BitMask=0xFF  BitMaskRealWorld=Stored Integer
  BitwiseOR{,1..3} (4 alike) : simulink/Logic and Bit Operations/Bitwise Operator  logicop=OR  UseBitMask=off  BitMask=bin2dec('11011001')  BitMaskRealWorld=Stored Integer
  BitwiseOR4 : simulink/Logic and Bit Operations/Bitwise Operator  logicop=OR  UseBitMask=off  NumInputPorts=8  BitMask=bin2dec('11011001')  BitMaskRealWorld=Stored Integer
  ChecksumABM1 : Subsystem
  CrashOutputSts : Subsystem
  DDM_CS&RC_Comparison : FVT_lib/hal/DDM_CS&RC_Comparison  MsgCycleTime=500
  Data Type Conversion{,1..11} (12 alike) : DataTypeConversion  OutDataTypeStr=uint8
  DriverSeatBeltCmd : Subsystem
  KHAL_CAN1ABM1E2E_flg : Constant  Value=KHAL_CAN1ABM1E2E_flg
  LeftShift{,1..2,11} (4 alike) : ArithShift  BitShiftDirection=Left
  LeftShift10 : ArithShift  BitShiftNumber=7  BitShiftDirection=Left
  LeftShift3 : ArithShift  BitShiftNumber=1  BitShiftDirection=Left
  LeftShift4 : ArithShift  BitShiftNumber=4  BitShiftDirection=Left
  LeftShift5 : ArithShift  BitShiftNumber=3  BitShiftDirection=Left
  LeftShift6 : ArithShift  BitShiftNumber=2  BitShiftDirection=Left
  LeftShift7 : ArithShift  BitShiftNumber=6  BitShiftDirection=Left
  LeftShift8 : ArithShift  BitShiftNumber=4  BitShiftDirection=Left
  LeftShift9 : ArithShift  BitShiftNumber=5  BitShiftDirection=Left
  LifeCountABM1 : Subsystem
  MessageRollingCounter : FVT_lib/hal/MessageRollingCounter  CounterMAX=14  task_time_ms=5  msg_time_ms=500
  Mux : Mux  Inputs=7
  PsngrSeatBeltCmd : Subsystem
  RCenterSeatBeltCmd : Subsystem
  RDriverSeatBeltCmd : Subsystem
  RPsngrSeatBeltCmd : Subsystem
  bus_selector : BusSelector  OutputSignals=CAN1_AirBagFailCmd,CAN1_Checksum_ABM1,CAN1_CrashOutputSts,CAN1_DriverSeatBeltCmd,CAN1_LifeCount_ABM1,CAN1_PABSwitchCmd,CAN1_PsngrSeatBeltCmd,CAN1_RCenterSeatBeltCmd,CAN1_RDriverSeatBeltCmd,CAN1_RPsngrSeatBeltCmd,CAN1_TLHPsngrSeatBeltCmd,CAN1_TRHPsngrSeatBeltCmd
  bus_selector1 : BusSelector  OutputSignals=CAN1_AirBagFailCmd
  bus_selector2 : BusSelector  OutputSignals=CAN1_Checksum_ABM1
  bus_selector3 : BusSelector  OutputSignals=CAN1_CrashOutputSts
  bus_selector4 : BusSelector  OutputSignals=CAN1_DriverSeatBeltCmd
  bus_selector5 : BusSelector  OutputSignals=CAN1_LifeCount_ABM1
  bus_selector6 : BusSelector  OutputSignals=CAN1_PsngrSeatBeltCmd
  bus_selector7 : BusSelector  OutputSignals=CAN1_RCenterSeatBeltCmd
  bus_selector8 : BusSelector  OutputSignals=CAN1_RDriverSeatBeltCmd
  bus_selector9 : BusSelector  OutputSignals=CAN1_RPsngrSeatBeltCmd
  constant : Constant  Value=0x0  OutDataTypeStr=uint8
  constant1 : Constant  Value=0x0  OutDataTypeStr=uint8
  constant2 : Constant  Value=0x0  OutDataTypeStr=uint8
  VHAL_ABM1CSErr_flg : Outport
  VHAL_ABM1RCErr_flg : Outport  Port=2
  VHAL_AirBagFailCmd_flg : Outport  Port=3
  VHAL_ChecksumABM1_enum : Outport  Port=4
  VHAL_CrashOutputSts_enum : Outport  Port=5
  VHAL_DriverSeatBeltCmd_flg : Outport  Port=6
  VHAL_LifeCountABM1_enum : Outport  Port=7
  VHAL_PsngrSeatBeltCmd_flg : Outport  Port=8
  VHAL_RCenterSeatBeltCmd_flg : Outport  Port=9
  VHAL_RDriverSeatBeltCmd_flg : Outport  Port=10
  VHAL_RPsngrSeatBeltCmd_flg : Outport  Port=11
  wires:
  DT_CAN1_SG_ABM1/1 -> [DT_CAN1_SG_ABM1]
  [DT_CAN1_SG_ABM1] -> bus_selector/1
  bus_selector/1 -> [CAN1_AirBagFailCmd]  "<CAN1_AirBagFailCmd>"
  [CAN1_AirBagFailCmd] -> LeftShift/1
  LeftShift/1 -> BitwiseAND/1
  BitwiseAND/1 -> [Byte_7_CAN1_AirBagFailCmd]
  bus_selector/2 -> [CAN1_Checksum_ABM1]  "<CAN1_Checksum_ABM1>"
  [CAN1_Checksum_ABM1] -> LeftShift1/1
  LeftShift1/1 -> BitwiseAND1/1
  BitwiseAND1/1 -> [Byte_0_CAN1_Checksum_ABM1]
  bus_selector/3 -> [CAN1_CrashOutputSts]  "<CAN1_CrashOutputSts>"
  [CAN1_CrashOutputSts] -> LeftShift2/1
  LeftShift2/1 -> BitwiseAND2/1
  BitwiseAND2/1 -> [Byte_5_CAN1_CrashOutputSts]
  bus_selector/4 -> [CAN1_DriverSeatBeltCmd]  "<CAN1_DriverSeatBeltCmd>"
  [CAN1_DriverSeatBeltCmd] -> LeftShift3/1
  LeftShift3/1 -> BitwiseAND3/1
  BitwiseAND3/1 -> [Byte_7_CAN1_DriverSeatBeltCmd]
  bus_selector/5 -> [CAN1_LifeCount_ABM1]  "<CAN1_LifeCount_ABM1>"
  [CAN1_LifeCount_ABM1] -> LeftShift4/1
  LeftShift4/1 -> BitwiseAND4/1
  BitwiseAND4/1 -> [Byte_1_CAN1_LifeCount_ABM1]
  bus_selector/6 -> [CAN1_PABSwitchCmd]  "<CAN1_PABSwitchCmd>"
  [CAN1_PABSwitchCmd] -> LeftShift5/1
  LeftShift5/1 -> BitwiseAND5/1
  BitwiseAND5/1 -> [Byte_7_CAN1_PABSwitchCmd]
  bus_selector/7 -> [CAN1_PsngrSeatBeltCmd]  "<CAN1_PsngrSeatBeltCmd>"
  [CAN1_PsngrSeatBeltCmd] -> LeftShift6/1
  LeftShift6/1 -> BitwiseAND6/1
  BitwiseAND6/1 -> [Byte_7_CAN1_PsngrSeatBeltCmd]
  bus_selector/8 -> [CAN1_RCenterSeatBeltCmd]  "<CAN1_RCenterSeatBeltCmd>"
  [CAN1_RCenterSeatBeltCmd] -> LeftShift7/1
  LeftShift7/1 -> BitwiseAND7/1
  BitwiseAND7/1 -> [Byte_7_CAN1_RCenterSeatBeltCmd]
  bus_selector/9 -> [CAN1_RDriverSeatBeltCmd]  "<CAN1_RDriverSeatBeltCmd>"
  [CAN1_RDriverSeatBeltCmd] -> LeftShift8/1
  LeftShift8/1 -> BitwiseAND8/1
  BitwiseAND8/1 -> [Byte_7_CAN1_RDriverSeatBeltCmd]
  bus_selector/10 -> [CAN1_RPsngrSeatBeltCmd]  "<CAN1_RPsngrSeatBeltCmd>"
  [CAN1_RPsngrSeatBeltCmd] -> LeftShift9/1
  LeftShift9/1 -> BitwiseAND9/1
  BitwiseAND9/1 -> [Byte_7_CAN1_RPsngrSeatBeltCmd]
  bus_selector/11 -> [CAN1_TLHPsngrSeatBeltCmd]  "<CAN1_TLHPsngrSeatBeltCmd>"
  [CAN1_TLHPsngrSeatBeltCmd] -> LeftShift10/1
  LeftShift10/1 -> BitwiseAND10/1
  BitwiseAND10/1 -> [Byte_7_CAN1_TLHPsngrSeatBeltCmd]
  bus_selector/12 -> [CAN1_TRHPsngrSeatBeltCmd]  "<CAN1_TRHPsngrSeatBeltCmd>"
  [CAN1_TRHPsngrSeatBeltCmd] -> LeftShift11/1
  LeftShift11/1 -> BitwiseAND11/1
  BitwiseAND11/1 -> [Byte_6_CAN1_TRHPsngrSeatBeltCmd]
  Data Type Conversion/1 -> BitwiseOR/1
  [Byte_0_CAN1_Checksum_ABM1] -> Data Type Conversion/1
  BitwiseOR/1 -> [Byte_0]
  Data Type Conversion1/1 -> BitwiseOR1/1
  [Byte_1_CAN1_LifeCount_ABM1] -> Data Type Conversion1/1
  BitwiseOR1/1 -> [Byte_1]
  constant/1 -> [Byte_2]
  constant1/1 -> [Byte_3]
  constant2/1 -> [Byte_4]
  Data Type Conversion2/1 -> BitwiseOR2/1
  [Byte_5_CAN1_CrashOutputSts] -> Data Type Conversion2/1
  BitwiseOR2/1 -> [Byte_5]
  Data Type Conversion3/1 -> BitwiseOR3/1
  [Byte_6_CAN1_TRHPsngrSeatBeltCmd] -> Data Type Conversion3/1
  BitwiseOR3/1 -> [Byte_6]
  Data Type Conversion4/1 -> BitwiseOR4/1
  [Byte_7_CAN1_AirBagFailCmd] -> Data Type Conversion4/1
  Data Type Conversion5/1 -> BitwiseOR4/2
  [Byte_7_CAN1_DriverSeatBeltCmd] -> Data Type Conversion5/1
  Data Type Conversion6/1 -> BitwiseOR4/3
  [Byte_7_CAN1_PABSwitchCmd] -> Data Type Conversion6/1
  Data Type Conversion7/1 -> BitwiseOR4/4
  [Byte_7_CAN1_PsngrSeatBeltCmd] -> Data Type Conversion7/1
  Data Type Conversion8/1 -> BitwiseOR4/5
  [Byte_7_CAN1_RCenterSeatBeltCmd] -> Data Type Conversion8/1
  Data Type Conversion9/1 -> BitwiseOR4/6
  [Byte_7_CAN1_RDriverSeatBeltCmd] -> Data Type Conversion9/1
  Data Type Conversion10/1 -> BitwiseOR4/7
  [Byte_7_CAN1_RPsngrSeatBeltCmd] -> Data Type Conversion10/1
  Data Type Conversion11/1 -> BitwiseOR4/8
  [Byte_7_CAN1_TLHPsngrSeatBeltCmd] -> Data Type Conversion11/1
  BitwiseOR4/1 -> [Byte_7]
  [Byte_1] -> Mux/1
  [Byte_2] -> Mux/2
  [Byte_3] -> Mux/3
  [Byte_4] -> Mux/4
  [Byte_5] -> Mux/5
  [Byte_6] -> Mux/6
  [Byte_7] -> Mux/7
  Mux/1 -> [VHAL_CAN1ABM1noCS_raw]
  KHAL_CAN1ABM1E2E_flg/1 -> DDM_CS&RC_Comparison/1
  0xf2/1 -> DDM_CS&RC_Comparison/2
  0xe4/1 -> DDM_CS&RC_Comparison/3
  [VHAL_CAN1ABM1noCS_raw] -> DDM_CS&RC_Comparison/4
  [Byte_0] -> DDM_CS&RC_Comparison/5
  [RC_ECU] -> DDM_CS&RC_Comparison/6
  MessageRollingCounter/1 -> DDM_CS&RC_Comparison/7
  DDM_CS&RC_Comparison/1 -> VHAL_ABM1CSErr_flg/1
  DDM_CS&RC_Comparison/2 -> VHAL_ABM1RCErr_flg/1
  [DT_CAN1_SG_ABM1] -> bus_selector1/1
  bus_selector1/1 -> AirBagFailCmd/1(AirBagFailCmd)  "<CAN1_AirBagFailCmd>"
  AirBagFailCmd/1(VHAL_AirBagFailCmd_flg) -> VHAL_AirBagFailCmd_flg/1
  [DT_CAN1_SG_ABM1] -> bus_selector2/1
  bus_selector2/1 -> ChecksumABM1/1(Checksum_ABM1)  "<CAN1_Checksum_ABM1>"
  ChecksumABM1/1(VHAL_ChecksumABM1_enum) -> VHAL_ChecksumABM1_enum/1
  [DT_CAN1_SG_ABM1] -> bus_selector3/1
  bus_selector3/1 -> CrashOutputSts/1(CrashOutputSts)  "<CAN1_CrashOutputSts>"
  CrashOutputSts/1(VHAL_CrashOutputSts_enum) -> VHAL_CrashOutputSts_enum/1
  [DT_CAN1_SG_ABM1] -> bus_selector4/1
  bus_selector4/1 -> DriverSeatBeltCmd/1(DriverSeatBeltCmd)  "<CAN1_DriverSeatBeltCmd>"
  DriverSeatBeltCmd/1(VHAL_DriverSeatBeltCmd_flg) -> VHAL_DriverSeatBeltCmd_flg/1
  [DT_CAN1_SG_ABM1] -> bus_selector5/1
  bus_selector5/1 -> LifeCountABM1/1(LifeCount_ABM1)  "<CAN1_LifeCount_ABM1>"
  LifeCountABM1/1(VHAL_LifeCountABM1_enum) -> VHAL_LifeCountABM1_enum/1, [RC_ECU]
  [DT_CAN1_SG_ABM1] -> bus_selector6/1
  bus_selector6/1 -> PsngrSeatBeltCmd/1(PsngrSeatBeltCmd)  "<CAN1_PsngrSeatBeltCmd>"
  PsngrSeatBeltCmd/1(VHAL_PsngrSeatBeltCmd_flg) -> VHAL_PsngrSeatBeltCmd_flg/1
  [DT_CAN1_SG_ABM1] -> bus_selector7/1
  bus_selector7/1 -> RCenterSeatBeltCmd/1(RCenterSeatBeltCmd)  "<CAN1_RCenterSeatBeltCmd>"
  RCenterSeatBeltCmd/1(VHAL_RCenterSeatBeltCmd_flg) -> VHAL_RCenterSeatBeltCmd_flg/1
  [DT_CAN1_SG_ABM1] -> bus_selector8/1
  bus_selector8/1 -> RDriverSeatBeltCmd/1(RDriverSeatBeltCmd)  "<CAN1_RDriverSeatBeltCmd>"
  RDriverSeatBeltCmd/1(VHAL_RDriverSeatBeltCmd_flg) -> VHAL_RDriverSeatBeltCmd_flg/1
  [DT_CAN1_SG_ABM1] -> bus_selector9/1
  bus_selector9/1 -> RPsngrSeatBeltCmd/1(RPsngrSeatBeltCmd)  "<CAN1_RPsngrSeatBeltCmd>"
  RPsngrSeatBeltCmd/1(VHAL_RPsngrSeatBeltCmd_flg) -> VHAL_RPsngrSeatBeltCmd_flg/1

== system halin/HAL_IN/CAN1/EPAS1 ==
  DT_CAN1_SG_EPAS1 : Inport
  DriIntend : Subsystem
  EPSAOIControl : Subsystem
  bus_selector : BusSelector  OutputSignals=CAN1_DriIntend
  bus_selector1 : BusSelector  OutputSignals=CAN1_EPS_AOI_Control
  VHAL_DriIntend_enum : Outport
  VHAL_EPSAOIControl_enum : Outport  Port=2
  wires:
  DT_CAN1_SG_EPAS1/1 -> [DT_CAN1_SG_EPAS1]
  [DT_CAN1_SG_EPAS1] -> bus_selector/1
  bus_selector/1 -> DriIntend/1(DriIntend)  "<CAN1_DriIntend>"
  DriIntend/1(VHAL_DriIntend_enum) -> VHAL_DriIntend_enum/1
  [DT_CAN1_SG_EPAS1] -> bus_selector1/1
  bus_selector1/1 -> EPSAOIControl/1(EPS_AOI_Control)  "<CAN1_EPS_AOI_Control>"
  EPSAOIControl/1(VHAL_EPSAOIControl_enum) -> VHAL_EPSAOIControl_enum/1

== system halin/HAL_IN/CAN1/EPAS2 ==
  DT_CAN1_SG_EPAS2 : Inport
  SASAngle : Subsystem
  SASCAL : Subsystem
  SASSpeed : Subsystem
  SASSpeedValid : Subsystem
  SASV : Subsystem
  bus_selector : BusSelector  OutputSignals=CAN1_SAS_Angle
  bus_selector1 : BusSelector  OutputSignals=CAN1_SAS_CAL
  bus_selector2 : BusSelector  OutputSignals=CAN1_SAS_Speed
  bus_selector3 : BusSelector  OutputSignals=CAN1_SAS_Speed_Valid
  bus_selector4 : BusSelector  OutputSignals=CAN1_SAS_V
  VHAL_SASAngle_Deg : Outport
  VHAL_SASCAL_flg : Outport  Port=2
  VHAL_SASSpeed_degps : Outport  Port=3
  VHAL_SASSpeedValid_flg : Outport  Port=4
  VHAL_SASV_flg : Outport  Port=5
  wires:
  DT_CAN1_SG_EPAS2/1 -> [DT_CAN1_SG_EPAS2]
  [DT_CAN1_SG_EPAS2] -> bus_selector/1
  bus_selector/1 -> SASAngle/1(SAS_Angle)  "<CAN1_SAS_Angle>"
  SASAngle/1(VHAL_SASAngle_Deg) -> VHAL_SASAngle_Deg/1
  [DT_CAN1_SG_EPAS2] -> bus_selector1/1
  bus_selector1/1 -> SASCAL/1(SAS_CAL)  "<CAN1_SAS_CAL>"
  SASCAL/1(VHAL_SASCAL_flg) -> VHAL_SASCAL_flg/1
  [DT_CAN1_SG_EPAS2] -> bus_selector2/1
  bus_selector2/1 -> SASSpeed/1(SAS_Speed)  "<CAN1_SAS_Speed>"
  SASSpeed/1(VHAL_SASSpeed_degps) -> VHAL_SASSpeed_degps/1
  [DT_CAN1_SG_EPAS2] -> bus_selector3/1
  bus_selector3/1 -> SASSpeedValid/1(SAS_Speed_Valid)  "<CAN1_SAS_Speed_Valid>"
  SASSpeedValid/1(VHAL_SASSpeedValid_flg) -> VHAL_SASSpeedValid_flg/1
  [DT_CAN1_SG_EPAS2] -> bus_selector4/1
  bus_selector4/1 -> SASV/1(SAS_V)  "<CAN1_SAS_V>"
  SASV/1(VHAL_SASV_flg) -> VHAL_SASV_flg/1

== system halin/HAL_IN/CAN1/EPB1 ==
  DT_CAN1_SG_EPB1 : Inport
  DOASta : Subsystem
  EPBCarWashMode : Subsystem
  EPBErrSta : Subsystem
  EPBExtApplyAvail : Subsystem
  EPBExtReleaseAvail : Subsystem
  EPBSta : Subsystem
  bus_selector : BusSelector  OutputSignals=CAN1_DOA_Sta
  bus_selector1 : BusSelector  OutputSignals=CAN1_EPBCarWashMode
  bus_selector2 : BusSelector  OutputSignals=CAN1_EPBErrSta
  bus_selector3 : BusSelector  OutputSignals=CAN1_EPBExtApplyAvail
  bus_selector4 : BusSelector  OutputSignals=CAN1_EPBExtReleaseAvail
  bus_selector5 : BusSelector  OutputSignals=CAN1_EPBSta
  VHAL_DOASta_flg : Outport
  VHAL_EPBCarWashMode_flg : Outport  Port=2
  VHAL_EPBErrSta_enum : Outport  Port=3
  VHAL_EPBExtApplyAvail_flg : Outport  Port=4
  VHAL_EPBExtReleaseAvail_flg : Outport  Port=5
  VHAL_EPBSta_enum : Outport  Port=6
  wires:
  DT_CAN1_SG_EPB1/1 -> [DT_CAN1_SG_EPB1]
  [DT_CAN1_SG_EPB1] -> bus_selector/1
  bus_selector/1 -> DOASta/1(DOA_Sta)  "<CAN1_DOA_Sta>"
  DOASta/1(VHAL_DOASta_flg) -> VHAL_DOASta_flg/1
  [DT_CAN1_SG_EPB1] -> bus_selector1/1
  bus_selector1/1 -> EPBCarWashMode/1(EPBCarWashMode)  "<CAN1_EPBCarWashMode>"
  EPBCarWashMode/1(VHAL_EPBCarWashMode_flg) -> VHAL_EPBCarWashMode_flg/1
  [DT_CAN1_SG_EPB1] -> bus_selector2/1
  bus_selector2/1 -> EPBErrSta/1(EPBErrSta)  "<CAN1_EPBErrSta>"
  EPBErrSta/1(VHAL_EPBErrSta_enum) -> VHAL_EPBErrSta_enum/1
  [DT_CAN1_SG_EPB1] -> bus_selector3/1
  bus_selector3/1 -> EPBExtApplyAvail/1(EPBExtApplyAvail)  "<CAN1_EPBExtApplyAvail>"
  EPBExtApplyAvail/1(VHAL_EPBExtApplyAvail_flg) -> VHAL_EPBExtApplyAvail_flg/1
  [DT_CAN1_SG_EPB1] -> bus_selector4/1
  bus_selector4/1 -> EPBExtReleaseAvail/1(EPBExtReleaseAvail)  "<CAN1_EPBExtReleaseAvail>"
  EPBExtReleaseAvail/1(VHAL_EPBExtReleaseAvail_flg) -> VHAL_EPBExtReleaseAvail_flg/1
  [DT_CAN1_SG_EPB1] -> bus_selector5/1
  bus_selector5/1 -> EPBSta/1(EPBSta)  "<CAN1_EPBSta>"
  EPBSta/1(VHAL_EPBSta_enum) -> VHAL_EPBSta_enum/1
